simulink model "C2"  (R2024a)
settings: Solver=VariableStepAuto  StartTime=0.0  StopTime=10.0  RelTol=1e-3

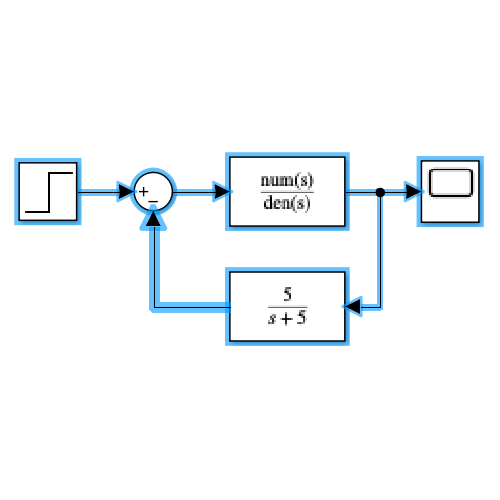
[thumbnail: Simulink's stored preview of the top-level diagram]
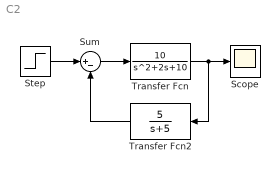
== system C2 ==
  Scope : Scope
  Step : Step  Time=0  After=2  SampleTime=0
  Sum : Sum  Inputs=|+-
  Transfer Fcn : TransferFcn  Numerator=[10]  Denominator=[1 2 10]
  Transfer Fcn2 : TransferFcn  Numerator=[5]  Denominator=[1 5]
  wires:
  Step/1 -> Sum/1
  Transfer Fcn/1 -> Scope/1, Transfer Fcn2/1
  Sum/1 -> Transfer Fcn/1
  Transfer Fcn2/1 -> Sum/2
